simulink model "Feedback_Control"  (R2025a)
settings: Solver=VariableStepAuto  StartTime=0.0  StopTime=100  RelTol=1e-3
undefined symbols (not defined in the file or in its folder): B, J, K, Ki, Kp
settings Model: Creator=yurru  LastModifiedBy=yurru

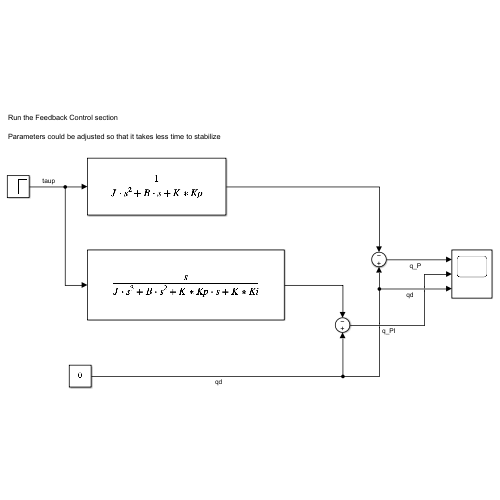
[thumbnail: Simulink's stored preview of the top-level diagram]
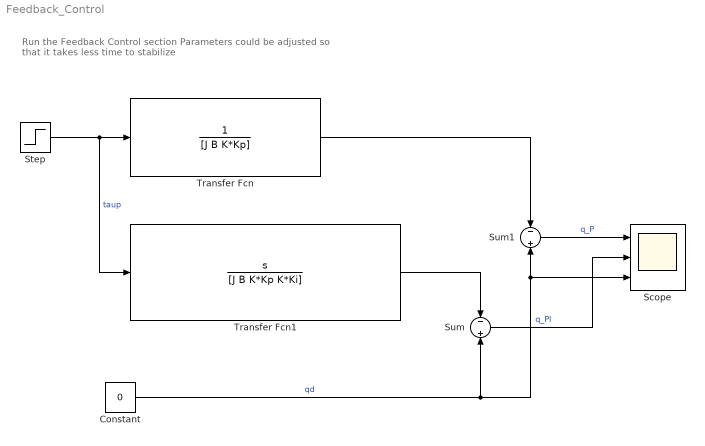
== system Feedback_Control ==
  note: Run the Feedback Control section
      |
      | Parameters could be adjusted so that it takes less time to stabilize
  Constant : Constant  Value=0
  Scope : Scope  NumInputPorts=3
      settings: ActiveDisplayYMinimum=-0.15798709157577154  ActiveDisplayYMaximum=0.09167236386183128
  Step : Step  SampleTime=0
  Sum : Sum  Inputs=-||+
  Sum1 : Sum  Inputs=-||+
  Transfer Fcn : TransferFcn  Denominator=[J B K*Kp]
  Transfer Fcn1 : TransferFcn  Numerator=[1 0]  Denominator=[J B K*Kp K*Ki]
  wires:
  Step/1 -> Transfer Fcn/1, Transfer Fcn1/1  "taup"
  Constant/1 -> Sum/2, Sum1/2, Scope/3  "qd"
  Transfer Fcn1/1 -> Sum/1
  Transfer Fcn/1 -> Sum1/1
  Sum1/1 -> Scope/1  "q_P"
  Sum/1 -> Scope/2  "q_PI"
